simulink model "kalman_filter"  (R2024b)
settings: Solver=VariableStepDiscrete  StartTime=0.0  StopTime=100.0  MaxStep=0.2  RelTol=1e-3
values from neighbouring files (symbols this model uses):
  P_0 = [100, 0, 0 ... (first row only)    [Workspace_Setup.m]
  Q_EKF = [0.0025, 0, 0 ... (first row only)    [Workspace_Setup.m]
  R_EKF = [1, 0 ... (first row only)    [Workspace_Setup.m]
  xhat_0 = [xhat_0_1 ... (first row only)    [Workspace_Setup.m]
settings Model: Creator=root  LastModifiedBy=root

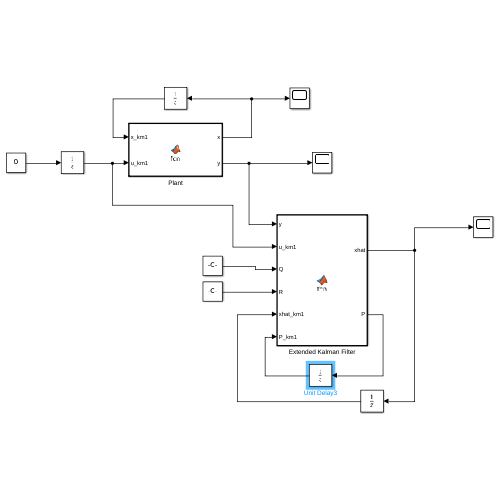
[thumbnail: Simulink's stored preview of the top-level diagram]
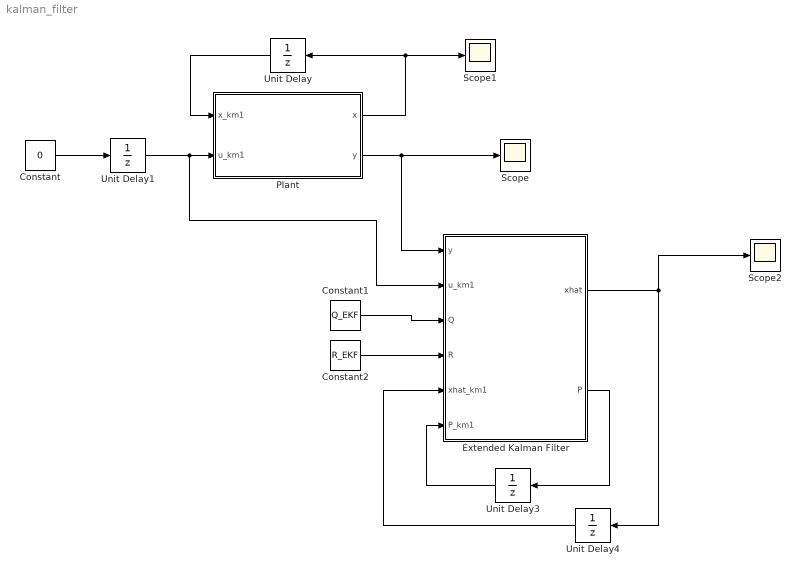
== system kalman_filter ==
  Constant : Constant  Value=0
  Constant1 : Constant  Value=Q_EKF
  Constant2 : Constant  Value=R_EKF
  Extended Kalman Filter : MATLAB Function  TreatAsAtomicUnit=on
  Plant : MATLAB Function  TreatAsAtomicUnit=on
  Scope : Scope
  Scope1 : Scope
  Scope2 : Scope
  Unit Delay : UnitDelay  InitialCondition=[5; 5; 0]  SampleTime=-1  HasFrameUpgradeWarning=on
  Unit Delay1 : UnitDelay  SampleTime=-1  HasFrameUpgradeWarning=on
  Unit Delay3 : UnitDelay  InitialCondition=P_0  SampleTime=-1  HasFrameUpgradeWarning=on
  Unit Delay4 : UnitDelay  InitialCondition=xhat_0  SampleTime=-1  HasFrameUpgradeWarning=on
  wires:
  Plant/1(x) -> Scope1/1, Unit Delay/1
  Unit Delay/1 -> Plant/1(x_km1)
  Constant/1 -> Unit Delay1/1
  Plant/2(y) -> Extended Kalman Filter/1(y), Scope/1
  Unit Delay1/1 -> Extended Kalman Filter/2(u_km1), Plant/2(u_km1)
  Extended Kalman Filter/2(P) -> Unit Delay3/1
  Unit Delay3/1 -> Extended Kalman Filter/6(P_km1)
  Unit Delay4/1 -> Extended Kalman Filter/5(xhat_km1)
  Constant1/1 -> Extended Kalman Filter/3(Q)
  Constant2/1 -> Extended Kalman Filter/4(R)
  Extended Kalman Filter/1(xhat) -> Scope2/1, Unit Delay4/1

== matlab function kalman_filter/Extended Kalman Filter ==
  data: y input; u_km1 input; Q input; R input; xhat output; xhat_km1 input; P_km1 input; P output; A parameter
function [xhat, P] = fcn(y, u_km1, Q, R, xhat_km1, P_km1, A)

% calculate predictions
xhat = [xhat_km1(1);
        xhat_km1(2) + xhat_km1(3);
        xhat_km1(3) + u_km1;];
yhat = [xhat(1)*cosd(xhat(2));
        xhat(1)*cosd(xhat(2) - xhat(3) + u_km1)];

% calculate new error covariance
P = A * P_km1 * A' + Q;
numerical_correction = [0.1, 0, 0;
                        0, 0.1, 0;
                        0, 0, 0.1;];
%P = P + numerical_correction;

% calculate C 
C11 = cosd(xhat(2));
C12 = -xhat(1) * sind(xhat(2));
C13 = 0;
C21 = cosd(xhat(2) - xhat(3) + u_km1);
C22 = -xhat(1) * sind(xhat(2) - xhat(3) + u_km1);
C23 = xhat(1) * sind(xhat(2) - xhat(3) + u_km1);
C = [C11, C12, C13;
       C21, C22, C23;];

% Calculate new Kalman gain
K = P * C' * inv(C * P * C' + R);

% Update prediction and covariance
xhat = xhat + K*(y-yhat);
P = (eye(3) - K*C)*P;

== matlab function kalman_filter/Plant ==
  data: x_km1 input; u_km1 input; x output; y output
% km1 = k minus 1
function [x, y] = fcn( x_km1, u_km1)

x1_km1 = x_km1(1);
x2_km1 = x_km1(2);
x3_km1 = x_km1(3);

x1 = x1_km1;
x2 = x2_km1 + x3_km1;
x3 = x3_km1 + u_km1;

y1 = x1*cosd(x2);
y2 = x1_km1*cosd(x2_km1);

x = [x1; x2; x3];
y = [y1; y2];
